simulink model "testEMS"  (R2018b)
settings: Solver=FixedStepAuto  StartTime=0.0  StopTime=420  FixedStep=1  RelTol=1e-3
settings Model: Creator=tortorod  LastModifiedBy=tortorod
settings DataIOCC: ExternalInput=[time, pload]  SaveOutput=off  SignalLogging=off  DSMLogging=off  SaveTime=off

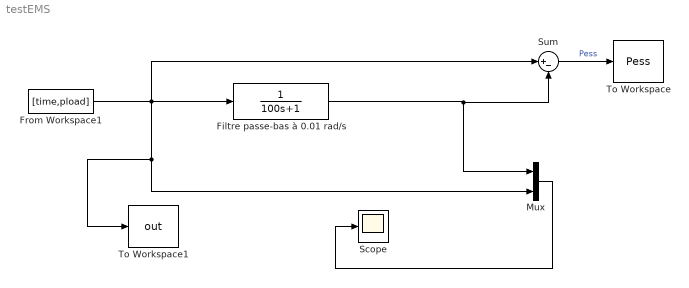
== system testEMS ==
  Filtre passe-bas à 0.01 rad/s : TransferFcn  Denominator=[100 1]
  From Workspace1 : FromWorkspace  VariableName=[time,pload]
  Mux : Mux  Inputs=2
  Scope : Scope
  Sum : Sum  Inputs=|+-
  To Workspace : ToWorkspace  VariableName=Pess  SaveFormat=Structure  SampleTime=-1
      settings: Save2DSignal=2-D array (concatenate along first dimension)
  To Workspace1 : ToWorkspace  VariableName=out  SaveFormat=Structure  SampleTime=-1
      settings: Save2DSignal=2-D array (concatenate along first dimension)
  wires:
  Filtre passe-bas à 0.01 rad/s/1 -> Sum/2, Mux/1
  Mux/1 -> Scope/1
  Sum/1 -> To Workspace/1  "Pess"
  From Workspace1/1 -> Sum/1, To Workspace1/1, Mux/2, Filtre passe-bas à 0.01 rad/s/1
